simulink model "RISE_virtualTest"  (R2018b)
settings: Solver=ode45  StartTime=0.0  StopTime=60  MaxStep=1e-3  RelTol=1e-3  AbsTol=1e-4
values from neighbouring files (symbols this model uses):
  W_hat_0 = 0.1*(rand(ctr_params.L,2)-0.5)    [RISE_params.m]    (also in RISE_virtualTest_params.m)
  x_0 = zeros(8,1)    [RISE_params.m]    (also in RISE_virtualTest_params.m = zeros(4,1))
settings Model: Creator=RUZHOU  LastModifiedBy=RUZHOU

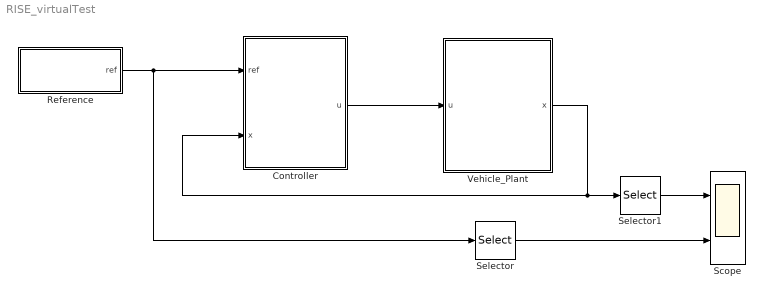
== system RISE_virtualTest ==
  Controller : Subsystem
  Reference : Subsystem
  Scope : Scope  NumInputPorts=2
  Selector : Selector  InputPortWidth=8  IndexOptions=Index vector (dialog)  Indices=[1 2]  OutputSizes=1
  Selector1 : Selector  InputPortWidth=4  IndexOptions=Index vector (dialog)  Indices=[1 2]  OutputSizes=1
  Vehicle_Plant : Subsystem
  wires:
  Controller/1(u) -> Vehicle_Plant/1(u)
  Reference/1(ref) -> Selector/1, Controller/1(ref)
  Vehicle_Plant/1(x) -> Selector1/1, Controller/2(x)
  Selector/1 -> Scope/2
  Selector1/1 -> Scope/1

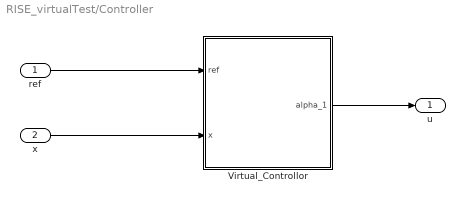
== system RISE_virtualTest/Controller ==
  ref : Inport
  x : Inport  Port=2
  Virtual_Controllor : Subsystem
  u : Outport
  wires:
  ref/1 -> Virtual_Controllor/1(ref)
  x/1 -> Virtual_Controllor/2(x)
  Virtual_Controllor/1(alpha_1) -> u/1

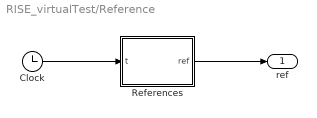
== system RISE_virtualTest/Reference ==
  Clock : Clock
  References : MATLAB Function  TreatAsAtomicUnit=on
  ref : Outport
  wires:
  Clock/1 -> References/1(t)
  References/1(ref) -> ref/1

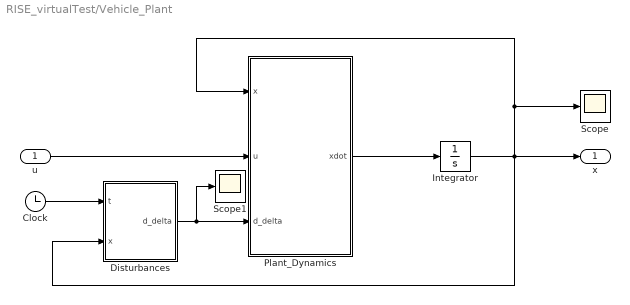
== system RISE_virtualTest/Vehicle_Plant ==
  u : Inport
  Clock : Clock
  Disturbances : MATLAB Function  TreatAsAtomicUnit=on
  Integrator : Integrator  InitialCondition=x_0
  Plant_Dynamics : MATLAB Function  TreatAsAtomicUnit=on
  Scope : Scope
  Scope1 : Scope
  x : Outport
  wires:
  Disturbances/1(d_delta) -> Scope1/1, Plant_Dynamics/3(d_delta)
  Clock/1 -> Disturbances/1(t)
  u/1 -> Plant_Dynamics/2(u)
  Plant_Dynamics/1(xdot) -> Integrator/1
  Integrator/1 -> Disturbances/2(x), Scope/1, Plant_Dynamics/1(x), x/1

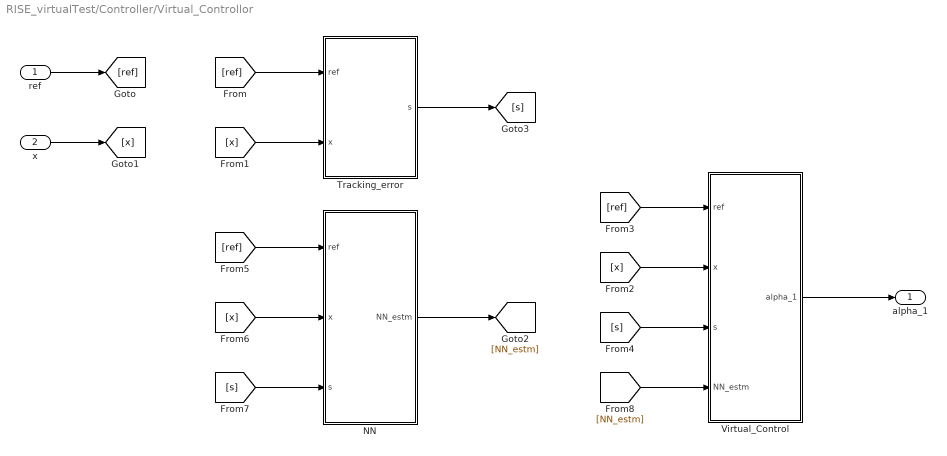
== system RISE_virtualTest/Controller/Virtual_Controllor ==
  ref : Inport
  x : Inport  Port=2
  NN : Subsystem
  Tracking_error : Subsystem
  Virtual_Control : Subsystem
  alpha_1 : Outport
  wires:
  [ref] -> Virtual_Control/1(ref)
  x/1 -> [x]
  ref/1 -> [ref]
  NN/1(NN_estm) -> [NN_estm]
  [NN_estm] -> Virtual_Control/4(NN_estm)
  [x] -> Virtual_Control/2(x)
  [x] -> NN/2(x)
  [s] -> NN/3(s)
  Tracking_error/1(s) -> [s]
  [s] -> Virtual_Control/3(s)
  [x] -> Tracking_error/2(x)
  [ref] -> Tracking_error/1(ref)
  [ref] -> NN/1(ref)
  Virtual_Control/1(alpha_1) -> alpha_1/1

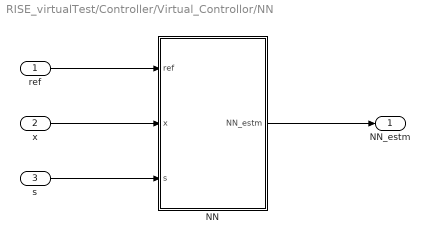
== system RISE_virtualTest/Controller/Virtual_Controllor/NN ==
  ref : Inport
  x : Inport  Port=2
  s : Inport  Port=3
  NN : Subsystem
  NN_estm : Outport
  wires:
  ref/1 -> NN/1(ref)
  x/1 -> NN/2(x)
  s/1 -> NN/3(s)
  NN/1(NN_estm) -> NN_estm/1

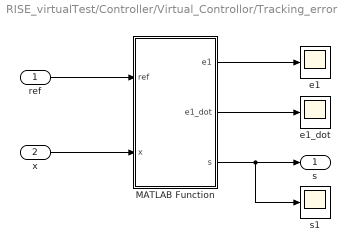
== system RISE_virtualTest/Controller/Virtual_Controllor/Tracking_error ==
  ref : Inport
  x : Inport  Port=2
  MATLAB Function : MATLAB Function  TreatAsAtomicUnit=on
  e1 : Scope
  e1_dot : Scope
  s1 : Scope
  s : Outport
  wires:
  MATLAB Function/2(e1_dot) -> e1_dot/1
  ref/1 -> MATLAB Function/1(ref)
  x/1 -> MATLAB Function/2(x)
  MATLAB Function/3(s) -> s1/1, s/1
  MATLAB Function/1(e1) -> e1/1

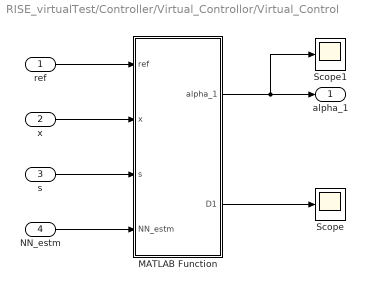
== system RISE_virtualTest/Controller/Virtual_Controllor/Virtual_Control ==
  ref : Inport
  x : Inport  Port=2
  s : Inport  Port=3
  NN_estm : Inport  Port=4
  MATLAB Function : MATLAB Function  TreatAsAtomicUnit=on
  Scope : Scope
  Scope1 : Scope
  alpha_1 : Outport
  wires:
  NN_estm/1 -> MATLAB Function/4(NN_estm)
  s/1 -> MATLAB Function/3(s)
  x/1 -> MATLAB Function/2(x)
  ref/1 -> MATLAB Function/1(ref)
  MATLAB Function/1(alpha_1) -> Scope1/1, alpha_1/1
  MATLAB Function/2(D1) -> Scope/1

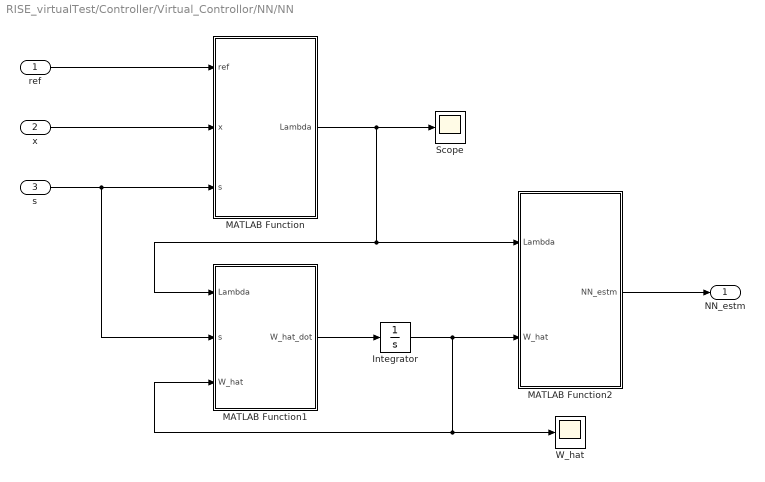
== system RISE_virtualTest/Controller/Virtual_Controllor/NN/NN ==
  ref : Inport
  x : Inport  Port=2
  s : Inport  Port=3
  Integrator : Integrator  InitialCondition=W_hat_0
  MATLAB Function : MATLAB Function  TreatAsAtomicUnit=on
  MATLAB Function1 : MATLAB Function  TreatAsAtomicUnit=on
  MATLAB Function2 : MATLAB Function  TreatAsAtomicUnit=on
  Scope : Scope
  W_hat : Scope
  NN_estm : Outport
  wires:
  x/1 -> MATLAB Function/2(x)
  s/1 -> MATLAB Function/3(s), MATLAB Function1/2(s)
  ref/1 -> MATLAB Function/1(ref)
  MATLAB Function/1(Lambda) -> Scope/1, MATLAB Function1/1(Lambda), MATLAB Function2/1(Lambda)
  MATLAB Function1/1(W_hat_dot) -> Integrator/1
  Integrator/1 -> MATLAB Function1/3(W_hat), W_hat/1, MATLAB Function2/2(W_hat)
  MATLAB Function2/1(NN_estm) -> NN_estm/1

== matlab function RISE_virtualTest/Vehicle_Plant/Disturbances ==
  data: t input; d_delta output size=2; x input size=4
function d_delta = fcn(t,x)
% states
x1 = x(1:2);
d = 1*([5e4;2e5]*exp(-2*t)*sin(6*t)+1*exp(-2*t)*x1);
d_delta = d;
end

== matlab function RISE_virtualTest/Vehicle_Plant/Plant_Dynamics ==
  data: x input size=4; u input size=2; xdot output size=4; d_delta input size=2; sys_params parameter
function xdot = fcn(x,u,d_delta,sys_params)
% Parameters
G1 = sys_params.G1;
n1 = sys_params.n1;
s1 = sys_params.s1;
G2 = sys_params.G2;
n2 = sys_params.n2;
s2 = sys_params.s2;
eta = sys_params.eta;
l = sys_params.l;
L1 = sys_params.L1;
L2 = sys_params.L2;
L3 = sys_params.L3;
L4 = sys_params.L4;
m2 = sys_params.m2;
theta_1 = sys_params.theta_1;
theta_2 = sys_params.theta_2;
theta_3 = sys_params.theta_3;
C = sys_params.C;
g = sys_params.g;

%% States
x1 = x(1:2); x2 = x(3:4);

%% Disturbance
d = d_delta(1:2);

%% Nonlinear Functions
% Ma
Ma = zeros(2,2);
Ma(1,1) = 2547 + 5400*(sin(x1(2)))^2 - 2*sin(x1(2))*cos(x1(2)) + 224*(cos(x1(2)))^2;
Ma(1,2) = 2.8*sin(x1(2)) + 13.7*cos(x1(2));
Ma(2,1) = Ma(1,2);
Ma(2,2) = 5343;
% Mb
Mb = zeros(2,2);
Mb(1,2) = (10350*cos(x1(2))*sin(x1(2)) + 1.5*((cos(x1(2)))^2-(sin(x1(2)))^2))*x2(1)...
    - (13.7*sin(x1(2)) - 2.8*cos(x1(2)))*x2(2);
Mb(2,1) = -1/2*Mb(1,2);
Mb(2,2) = (1.5*cos(x1(2)) - 6.8*sin(x1(2)))*x2(1);
% W1
q0 = atan(L1/L2);
xp1 = sqrt(L3^2 + L1^2 + L2^2 - 2*L3*sqrt(L1^2+L2^2)*cos(x1(2)+q0));
h12 = L3*sqrt(L1^2+L2^2)*sin(x1(2)+q0)/xp1;
W1 = diag([G1/n1,2*pi*eta*G2/(n2*l)*h12]);
% W2
W2 = diag([G2,2*pi*eta*G2/l*h12]);
% W3
delta_q1 = u(1)/n1 - x1(1);
delta_q2 = u(2)/n2 - x1(2);
mu_1 = -2*s1*tanh(delta_q1/(2*s1));
mu_2 = -2*s2*tanh(delta_q2/(2*s2));
W3 = [mu_1;mu_2];
% Mg
Mg = [0;m2*g*L4*cos(x1(2))];

% phi
phi_1 = diag([tanh(C(1,1)*x2(1)),tanh(C(1,2)*x2(2))]);
phi_2 = diag([tanh(C(2,1)*x2(1))-tanh(C(3,1)*x2(1)),tanh(C(2,2)*x2(2))-tanh(C(3,2)*x2(2))]);
phi_3 = diag([x2(1),x2(2)]);
phi = [phi_1;phi_2;phi_3];
% theta
theta = [theta_1;theta_2;theta_3];

%% Dynamics
x1dot = x2;
x2dot = Ma\(W1*u - W2*x1 + W3 - Mb*x2 - (phi')*theta - Mg - d);


xdot = [x1dot;x2dot];
end

== matlab function RISE_virtualTest/Reference/References ==
  data: t input; ref output size=8
function ref = fcn(t)
% parameters
f1 = 0.1; a1 = 0.5; f2 = 0.15; a2 = 0.1;
x1d = [a1*sin(2*pi*f1*t);a2*sin(2*pi*f2*t)];
x1d_dot = [a1*2*pi*f1*cos(2*pi*f1*t);a2*2*pi*f2*cos(2*pi*f2*t)];
x1d_ddot = [-a1*(2*pi*f1)^2*sin(2*pi*f1*t);-a2*(2*pi*f2)^2*sin(2*pi*f2*t)];
x1d_3dot = [-a1*(2*pi*f1)^3*cos(2*pi*f1*t);-a2*(2*pi*f2)^3*cos(2*pi*f2*t)];
ref = [x1d;x1d_dot;x1d_ddot;x1d_3dot];
end

== matlab function RISE_virtualTest/Controller/Virtual_Controllor/NN/NN/MATLAB Function ==
  data: ref input size=8; Lambda output size=ctr_params.L; x input size=4; s input size=2; ctr_params parameter
function Lambda = fcn(ref,x,s,ctr_params)
% parameters
L = ctr_params.L;
c = ctr_params.c;
b = ctr_params.b;

% states
x1 = x(1:2); x2 = x(3:4);
x1d_dot = ref(3:4); x1d_ddot = ref(5:6);
e1_dot = x2 - x1d_dot;
Z = [x1;x2;e1_dot;x1d_ddot;s];
Z_bar = [Z;1];

%% Gaussian Function
Lambda = zeros(L,1);
for i = 1:length(Lambda)
    Lambda(i,1) = exp(-((Z_bar-c)')*(Z_bar-c)/(2*b(i)^2));
end


end

== matlab function RISE_virtualTest/Controller/Virtual_Controllor/NN/NN/MATLAB Function1 ==
  data: Lambda input size=ctr_params.L; W_hat_dot output size=[ctr_params.L,2]; s input size=2; W_hat input size=[ctr_params.L,2]; ctr_params parameter
function W_hat_dot = fcn(Lambda,s,W_hat,ctr_params)
% parameters
gamma = ctr_params.gamma;
Gamma = ctr_params.Gamma;
beta = ctr_params.beta;

% Weight Update Law
W_hat_dot = gamma*Gamma*(Lambda*(s') - beta*W_hat);
end

== matlab function RISE_virtualTest/Controller/Virtual_Controllor/NN/NN/MATLAB Function2 ==
  data: Lambda input size=ctr_params.L; NN_estm output size=2; W_hat input size=[ctr_params.L,2]
function NN_estm = fcn(Lambda,W_hat)

NN_estm = (W_hat')*Lambda;
end

== matlab function RISE_virtualTest/Controller/Virtual_Controllor/Tracking_error/MATLAB Function ==
  data: ref input size=8; e1 output size=2; x input size=4; e1_dot output size=2; s output size=2; ctr_params parameter
function [e1,e1_dot,s] = fcn(ref,x,ctr_params)
sigma_1 = ctr_params.sigma_1;
x1 = x(1:2); x2 = x(3:4);
x1d = ref(1:2); x1d_dot = ref(3:4);

e1 = x1 - x1d;
e1_dot = x2 - x1d_dot;
s = e1_dot + sigma_1*e1;
end

== matlab function RISE_virtualTest/Controller/Virtual_Controllor/Virtual_Control/MATLAB Function ==
  data: ref input size=8; alpha_1 output size=2; x input size=4; s input size=2; NN_estm input size=2; ctr_params parameter; D1 output
function [alpha_1,D1] = fcn(ref,x,s,NN_estm,ctr_params)
%% parameters
% Nonimal plant
G1 = ctr_params.G1;
n1 = ctr_params.n1;
% s1 = ctr_params.s1;
G2 = ctr_params.G2;
n2 = ctr_params.n2;
% s2 = ctr_params.s2;
eta = ctr_params.eta;
l = ctr_params.l;
L1 = ctr_params.L1;
L2 = ctr_params.L2;
L3 = ctr_params.L3;
L4 = ctr_params.L4;
m2 = ctr_params.m2;
theta_1 = ctr_params.theta_1;
theta_2 = ctr_params.theta_2;
theta_3 = ctr_params.theta_3;
C = ctr_params.C;
g = ctr_params.g;
% Virtual control
sigma_1 = ctr_params.sigma_1;
rho = ctr_params.rho;
Kc1 = ctr_params.Kc1;
epsilon = ctr_params.epsilon;

%% states
x1 = x(1:2); x2 = x(3:4);
x1d_dot = ref(3:4); x1d_ddot = ref(5:6);
e1_dot = x2 - x1d_dot;

%% Nominal functions
% Ma
Ma = zeros(2,2);
Ma(1,1) = 2547 + 5400*(sin(x1(2)))^2 - 2*sin(x1(2))*cos(x1(2)) + 224*(cos(x1(2)))^2;
Ma(1,2) = 2.8*sin(x1(2)) + 13.7*cos(x1(2));
Ma(2,1) = Ma(1,2);
Ma(2,2) = 5343;
% Mb
Mb = zeros(2,2);
Mb(1,2) = (10350*cos(x1(2))*sin(x1(2)) + 1.5*((cos(x1(2)))^2-(sin(x1(2)))^2))*x2(1)...
    - (13.7*sin(x1(2)) - 2.8*cos(x1(2)))*x2(2);
Mb(2,1) = -1/2*Mb(1,2);
Mb(2,2) = (1.5*cos(x1(2)) - 6.8*sin(x1(2)))*x2(1);
% W1
q0 = atan(L1/L2);
xp1 = sqrt(L3^2 + L1^2 + L2^2 - 2*L3*sqrt(L1^2+L2^2)*cos(x1(2)+q0));
h12 = L3*sqrt(L1^2+L2^2)*sin(x1(2)+q0)/xp1;
W1 = diag([G1/n1,2*pi*eta*G2/(n2*l)*h12]);
% W2
W2 = diag([G2,2*pi*eta*G2/l*h12]);
% Mg
Mg = [0;m2*g*L4*cos(x1(2))];
% phi
phi_1 = diag([tanh(C(1,1)*x2(1)),tanh(C(1,2)*x2(2))]);
phi_2 = diag([tanh(C(2,1)*x2(1))-tanh(C(3,1)*x2(1)),tanh(C(2,2)*x2(2))-tanh(C(3,2)*x2(2))]);
phi_3 = diag([x2(1),x2(2)]);
phi = [phi_1;phi_2;phi_3];
% theta
theta = [theta_1;theta_2;theta_3];

% Mw
Mw = W1\Ma;
% f1w
f1w = W1\(-W2*x1 - Mb*x2 - (phi')*theta - Mg);
% dMw_dt
dA11_dt = (5400*2*sin(x1(2))*cos(x1(2)) - 2*((cos(x1(2)))^2-(sin(x1(2)))^2) - 224*2*cos(x1(2))*sin(x1(2)))*x2(2);
dA12_dt = (2.8*cos(x1(2)) - 13.7*sin(x1(2)))*x2(2);
dA21_dt = dA12_dt;
dA22_dt = 0;
dxp1_dt = 1/2*(L3^2 + L1^2 + L2^2 - 2*L3*sqrt(L1^2+L2^2)*cos(x1(2)+q0))^(-1/2)*(2*L3*sqrt(L1^2+L2^2)*sin(x1(2)+q0))*x2(2);
dh12_dt = (L3*sqrt(L1^2+L2^2)*cos(x1(2)+q0)*x2(2)*xp1 - L3*sqrt(L1^2+L2^2)*sin(x1(2)+q0)*dxp1_dt)/(xp1^2);
dMw_dt = zeros(2,2);
dMw_dt(1,1) = n1/G1*dA11_dt;
dMw_dt(1,2) = n1/G1*dA12_dt;
dMw_dt(2,1) = l*n2/(2*pi*eta*G2)*(dA21_dt*h12-Ma(2,1)*dh12_dt)/(h12^2);
dMw_dt(2,2) = l*n2/(2*pi*eta*G2)*(dA22_dt*h12-Ma(2,2)*dh12_dt)/(h12^2);

F1 = f1w + Mw*(sigma_1*e1_dot-x1d_ddot) + 1/2*dMw_dt*s;

%% Contorl Law
alpha_1 = -F1 - Kc1*s - NN_estm - rho*tanh(s/epsilon);
D1 = det(W1);
end
